simulink model "TF_motor"  (R2023a)
settings: Solver=VariableStepAuto  StartTime=0.0  StopTime=10.0  RelTol=1e-3
settings Model: Creator=Admin  LastModifiedBy=Admin

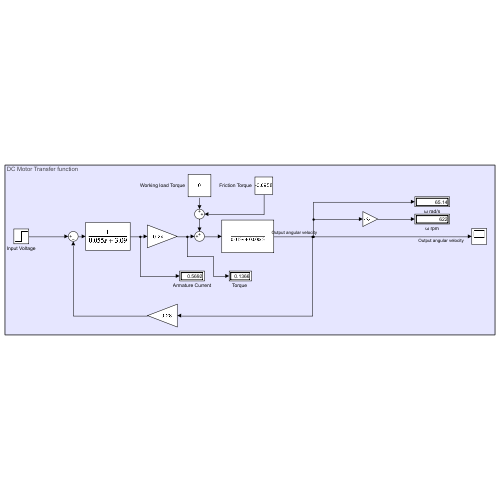
[thumbnail: Simulink's stored preview of the top-level diagram]
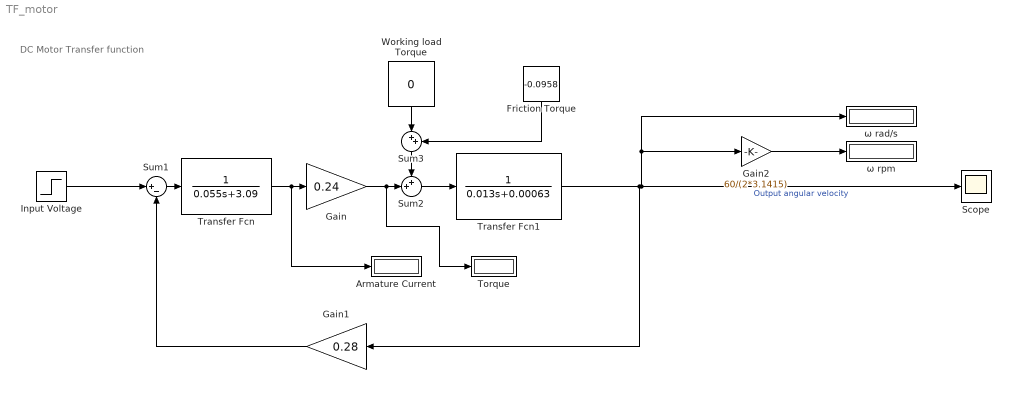
== system TF_motor ==
  note: DC Motor Transfer function
  Armature Current : Display
  Friction Torque : Constant  Value=-0.0958
  Gain : Gain  Gain=0.24
  Gain1 : Gain  Gain=0.28
  Gain2 : Gain  Gain=60/(2*3.1415)
  Input Voltage : Step  Time=0  After=20  SampleTime=0
  Scope : Scope
  Sum1 : Sum  Inputs=|+-
  Sum2 : Sum  Inputs=++|
  Sum3 : Sum  Inputs=|++
  "Torque " : Display
  Transfer Fcn : TransferFcn  Denominator=[0.055 3.09]
  Transfer Fcn1 : TransferFcn  Denominator=[0.013 0.00063]
  Working load Torque : Constant  Value=0
  ω rad/s : Display
  ω rpm : Display
  wires:
  Input Voltage/1 -> Sum1/1
  Gain1/1 -> Sum1/2
  Sum1/1 -> Transfer Fcn/1
  Transfer Fcn/1 -> Armature Current/1, Gain/1
  Gain2/1 -> ω rpm/1
  Sum2/1 -> Transfer Fcn1/1
  Gain/1 -> "Torque "/1, Sum2/2
  Transfer Fcn1/1 -> ω rad/s/1, Gain2/1, Scope/1, Gain1/1  "Output angular velocity"
  Sum3/1 -> Sum2/1
  Working load Torque/1 -> Sum3/1
  Friction Torque/1 -> Sum3/2
